simulink model "tempcon"  (R2020a)
settings: Solver=VariableStepAuto  StartTime=0.0  StopTime=100  RelTol=1e-3
settings Model: Creator=hp-pc  LastModifiedBy=hp-pc

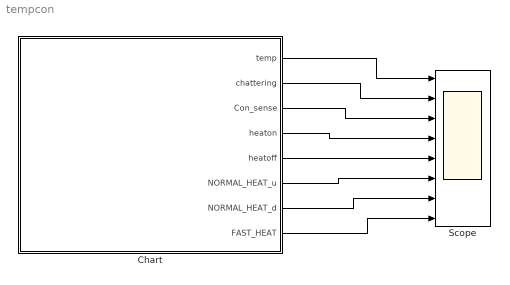
== system tempcon ==
  Chart : Stateflow chart  TreatAsAtomicUnit=on
      settings: PortSchema="{\"entries\":[{\"content\":{\"sides\":[{\"content\":{\"connectorIds\":[]},\"type\":\"ConnectorPlacement.EquallySpacedRectSide\",\"uuid\":\"c6a87a37-078d-45e8-a3e3-cabe2857dc14\"},{\"content\":{\"connectorIds\":[\"Out7\",\"Out8\",\"Out4\",\"Out6\",\"Out5\",\"Out2\",\"Out3\",\"Out1\"],\"side\":\"RIGHT\"},\"type\":\"ConnectorPlacement.EquallySpacedRectSide\",\"uuid\":\"e30d9a30-9c68-4d81-be3e-0648123adae3\"},{\"content\":{\"connectorIds\":[],\"side\":\"TOP\"},\"type\":\"ConnectorPlacement.EquallySpacedRectSide\",\"uuid\":\"c330568e-3be1-43c3-926a-465b61299a17\"}]},\"type\":\"ConnectorPlacement.EquallySpacedConnector\",\"uuid\":\"cd520344-a9e4-4f14-a072-999ed067088c\"}],\"packageUris\":[\"http://schema.mathworks.com/mf0/Connector/19700101\"],\"version\":\"1.0\"}"
  Scope : Scope  NumInputPorts=8
  wires:
  Chart/7(temp) -> Scope/1
  Chart/8(chattering) -> Scope/2
  Chart/4(Con_sense) -> Scope/3
  Chart/6(heaton) -> Scope/4
  Chart/5(heatoff) -> Scope/5
  Chart/2(NORMAL_HEAT_u) -> Scope/6
  Chart/3(NORMAL_HEAT_d) -> Scope/7
  Chart/1(FAST_HEAT) -> Scope/8

== stateflow chart tempcon/Chart ==
  settings: updateMethod=DISCRETE  sampleTime=0.2
  state FAST_HEAT
    50<temp <66;
    Con_sense=2;%much low to create equi
    FAST_HEAT=2;
    temp;
    temp=temp+2;
    heaton=2;
    heatoff=0;
  state NORMAL_HEAT_u
    66<temp<70;
    Con_sense=1;%temp crossing limit 70 high
    NORMAL_HEAT_u=1;
    FAST_HEAT=0;
    NORMAL_HEAT_d=0;
    heaton=1;
    heatoff=0;
    temp=temp+1;
    FAST_HEAT=0;
    %c;
    %c=c+1;
  state Controller_check
    temp=50;
    55< temp <75;
    temp=temp+1;
    %temp;
    Con_sense=0;
    FAST_HEAT=0;
    NORMAL_HEAT_u=0;
    NORMAL_HEAT_d=0;
    heaton=1;
    heatoff=0;
    Con_sense=1;
    c1=0;
    c2=0;
    %c=c+1;
    FAST_HEAT=0;
  note: initial 55° to 75° F and controller mode is OFF
      |
      | NORMAL_HEAT m-M
      | MAX_Temp 70 above on   heatoff
      | MIN_Temp 66 below off    heaton
      |
      | FAST_HEAT lower than MIN_Temp
      |
      | consecutively switches operation mode more than CHATTERING_LIMIT(2) ,
      | then it continues operating in previous mode without switching till next 5 sampling duration.
  note: 50<
  state NORMAL_HEAT_d%only dec below 70 if high
    60<temp <75;
    Con_sense=-1;%low till 66
    NORMAL_HEAT_d=-1;
    FAST_HEAT=0;
    NORMAL_HEAT_u=0;
    heatoff=1;
    heaton=0;
    temp=temp-1;
  state chattering
    %chattering=1;
    c1=0;
    c2=0;
  note: at(7,tick)[temp > 98.6]
  FAST_HEAT -> NORMAL_HEAT_u : [(temp>66)]%NORMAL mode above 66 heat on temp up
  Controller_check -> FAST_HEAT [order 3] : [(temp <66)&&(Con_sense==1)]%temp below 66 FAST mode
  Controller_check -> NORMAL_HEAT_u [order 1] : [(66==temp)&&(Con_sense==1)]
  (default) -> Controller_check
  NORMAL_HEAT_d%only dec below 70 if high -> NORMAL_HEAT_u [order 1] : [66>=temp]{c1=c1+1;}%check for below 50-66
  NORMAL_HEAT_u -> NORMAL_HEAT_d%only dec below 70 if high [order 1] : [temp>=70]{c2=c2+1;}%heat off temp down below 70
  NORMAL_HEAT_u -> chattering [order 2] : [c1==2]{c1=0;chattering=1;}
  chattering -> NORMAL_HEAT_u [order 2] : after(1,sec)[c1==0]{chattering=0;}
  Controller_check -> NORMAL_HEAT_d%only dec below 70 if high [order 2] : [(70<temp)&&(Con_sense==1)]
  NORMAL_HEAT_d%only dec below 70 if high -> chattering [order 2] : [c2==2]{c2=0;chattering=1;}
  chattering -> NORMAL_HEAT_d%only dec below 70 if high [order 1] : after(1,sec)[c2==0]{chattering=0;}
  data: FAST_HEAT output; NORMAL_HEAT_u output; NORMAL_HEAT_d output; Con_sense output double; heatoff output; heaton output; c1 local; c2 local; temp output double; chattering output
